simulink model "MPC_FOC"  (R2021a)
settings: Solver=VariableStepAuto  StartTime=0.0  StopTime=2  RelTol=1e-3
undefined symbols (not defined in the file): C1, JL, JM, K1, sigbuilder_block
libraries: powerlib_extras x9, spsDCVoltageSourceLib x4, spsPermanentMagnetSynchronousMachineLib x4, spsUniversalBridgeLib x4, spspowerguiLib x4, simulink x3, spsVoltageMeasurementLib x3, pid_lib x1
(part 2 of 2)

== system MPC_FOC/FOC/SVPWM/XYZ Caculate ==
  Ualpha : Inport
  Ubeta : Inport  Port=2
  Ts : Inport  Port=3
  Udc : Inport  Port=4
  Add : Sum
  Add1 : Sum  Inputs=+-
  Gain : Gain  Gain=3/2
  Gain1 : Gain  Gain=sqrt(3)
  Gain2 : Gain  Gain=sqrt(3)/2
  Math Function : Math  Operator=reciprocal  SignedPower=on  SaturateOnIntegerOverflow=on
  Mux : Mux  Inputs=3
  Product{,1..3} (4 alike) : Product
  XYZ : Outport
  wires:
  Mux/1 -> XYZ/1
  Product2/1 -> Mux/2
  Add1/1 -> Product3/1
  Add/1 -> Product2/1
  Gain2/1 -> Add/1, Add1/1
  Gain/1 -> Add1/2, Add/2
  Product3/1 -> Mux/3
  Product/1 -> Product3/2, Product2/2, Product1/2
  Product1/1 -> Mux/1
  Gain1/1 -> Product1/1
  Math Function/1 -> Product/2
  Udc/1 -> Math Function/1
  Ts/1 -> Product/1
  Ubeta/1 -> Gain1/1, Gain2/1
  Ualpha/1 -> Gain/1

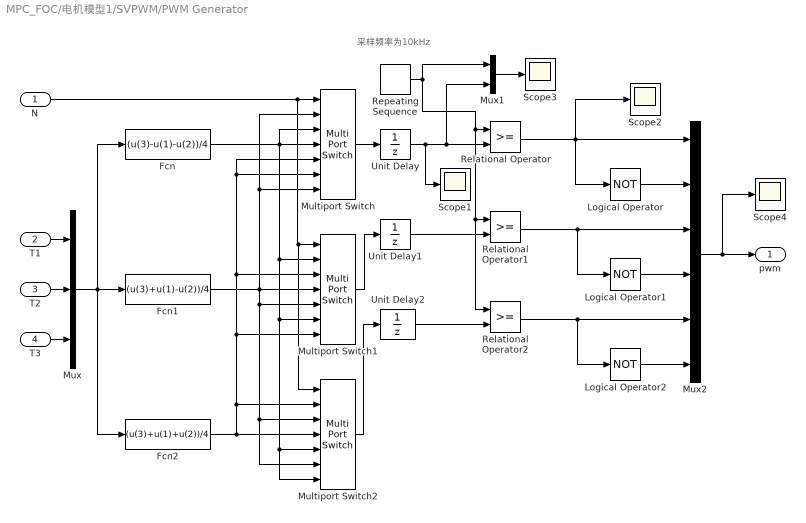
== system MPC_FOC/电机模型1/SVPWM/PWM Generator ==
  note: 采样频率为10kHz
  N : Inport
  T1 : Inport  Port=2
  T2 : Inport  Port=3
  T3 : Inport  Port=4
  Fcn : Fcn  Expr=(u(3)-u(1)-u(2))/4
  Fcn1 : Fcn  Expr=(u(3)+u(1)-u(2))/4
  Fcn2 : Fcn  Expr=(u(3)+u(1)+u(2))/4
  Logical Operator : Logic  Operator=NOT  AllPortsSameDT=off  OutDataTypeStr=boolean
  Logical Operator1 : Logic  Operator=NOT  AllPortsSameDT=off  OutDataTypeStr=boolean
  Logical Operator2 : Logic  Operator=NOT  AllPortsSameDT=off  OutDataTypeStr=boolean
  Multiport Switch : MultiPortSwitch  Inputs=6  DiagnosticForDefault=None
  Multiport Switch1 : MultiPortSwitch  Inputs=6  DiagnosticForDefault=None
  Multiport Switch2 : MultiPortSwitch  Inputs=6  DiagnosticForDefault=None
  Mux : Mux  Inputs=3
  Mux1 : Mux  Inputs=2
  Mux2 : Mux  Inputs=6
  Relational Operator : RelationalOperator  OutDataTypeStr=boolean  RndMeth=Nearest
  Relational Operator1 : RelationalOperator  OutDataTypeStr=boolean  RndMeth=Nearest
  Relational Operator2 : RelationalOperator  OutDataTypeStr=boolean  RndMeth=Nearest
  Repeating Sequence : simulink/Sources/Repeating Sequence  rep_seq_t=[0 0.00005 0.0001]  rep_seq_y=[0 0.00005 0]
  Scope{1..4} (4 alike) : Scope
  Unit Delay : UnitDelay  SampleTime=0.0001  HasFrameUpgradeWarning=on
  Unit Delay1 : UnitDelay  SampleTime=0.0001  HasFrameUpgradeWarning=on
  Unit Delay2 : UnitDelay  SampleTime=0.0001  HasFrameUpgradeWarning=on
  pwm : Outport
  wires:
  T2/1 -> Mux/2
  T1/1 -> Mux/1
  T3/1 -> Mux/3
  Mux/1 -> Fcn/1, Fcn1/1, Fcn2/1
  N/1 -> Multiport Switch2/1, Multiport Switch1/1, Multiport Switch/1
  Fcn/1 -> Multiport Switch2/7, Multiport Switch2/5, Multiport Switch1/6, Multiport Switch1/2, Multiport Switch/4, Multiport Switch/3
  Fcn1/1 -> Multiport Switch/7, Multiport Switch/2, Multiport Switch2/6, Multiport Switch2/3, Multiport Switch1/5, Multiport Switch1/4
  Fcn2/1 -> Multiport Switch2/4, Multiport Switch2/2, Multiport Switch1/7, Multiport Switch1/3, Multiport Switch/6, Multiport Switch/5
  Repeating Sequence/1 -> Mux1/1, Relational Operator2/1, Relational Operator1/1, Relational Operator/1
  Relational Operator/1 -> Scope2/1, Logical Operator/1, Mux2/1
  Relational Operator1/1 -> Logical Operator1/1, Mux2/3
  Relational Operator2/1 -> Logical Operator2/1, Mux2/5
  Logical Operator/1 -> Mux2/2
  Logical Operator1/1 -> Mux2/4
  Logical Operator2/1 -> Mux2/6
  Mux2/1 -> Scope4/1, pwm/1
  Multiport Switch1/1 -> Unit Delay1/1
  Multiport Switch2/1 -> Unit Delay2/1
  Multiport Switch/1 -> Unit Delay/1
  Mux1/1 -> Scope3/1
  Unit Delay/1 -> Mux1/2, Relational Operator/2, Scope1/1
  Unit Delay1/1 -> Relational Operator1/2
  Unit Delay2/1 -> Relational Operator2/2

== system MPC_FOC/电机模型1/SVPWM/Sector Caculate ==
  Ualpha : Inport
  "Ubeta " : Inport  Port=2
  Add : Sum  Inputs=+++
  Add1 : Sum  Inputs=+-
  Add2 : Sum  Inputs=--
  Constant : Constant
  Constant1 : Constant  Value=0
  Constant2 : Constant  Value=3/4
  Gain : Gain  Gain=4
  Gain1 : Gain  Gain=2
  Gain2 : Gain  Gain=0.5
  Product : Product
  Sqrt : Sqrt  SaturateOnIntegerOverflow=on
  Switch : Switch  Criteria=u2 > Threshold
  Switch1 : Switch  Criteria=u2 > Threshold
  Switch2 : Switch  Criteria=u2 > Threshold
  N : Outport
  wires:
  Ualpha/1 -> Product/1
  "Ubeta "/1 -> Switch/2, Gain2/1
  Add1/1 -> Switch1/2
  Add2/1 -> Switch2/2
  Constant/1 -> Switch/1, Switch1/1, Switch2/1
  Constant1/1 -> Switch2/3, Switch1/3, Switch/3
  Add/1 -> N/1
  Gain1/1 -> Add/2
  Gain/1 -> Add/3
  Switch2/1 -> Gain/1
  Switch1/1 -> Gain1/1
  Switch/1 -> Add/1
  Constant2/1 -> Sqrt/1
  Sqrt/1 -> Product/2
  Product/1 -> Add2/1, Add1/1
  Gain2/1 -> Add1/2, Add2/2

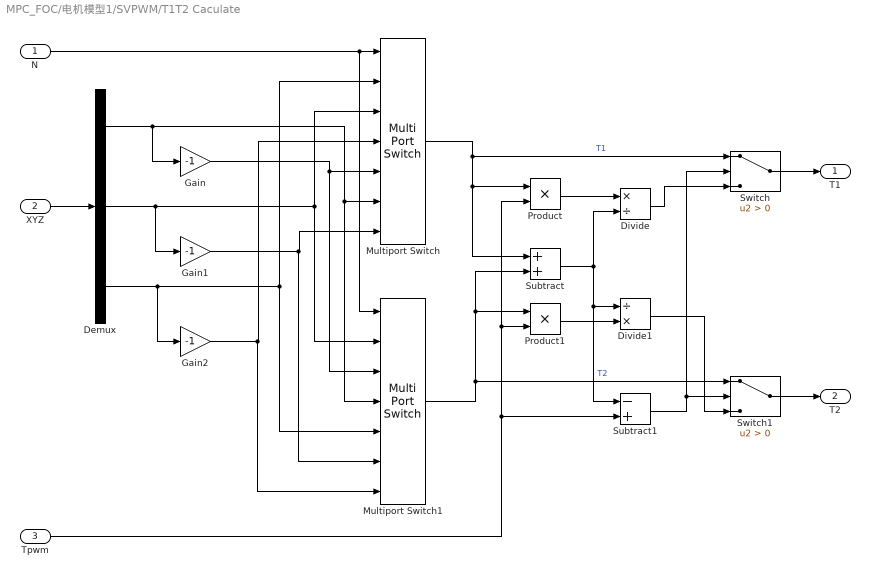
== system MPC_FOC/电机模型1/SVPWM/T1T2 Caculate ==
  N : Inport
  XYZ : Inport  Port=2
  Tpwm : Inport  Port=3
  Demux : Demux  Outputs=3
  Divide : Product  Inputs=*/
  Divide1 : Product  Inputs=/*
  Gain : Gain  Gain=-1
  Gain1 : Gain  Gain=-1
  Gain2 : Gain  Gain=-1
  Multiport Switch : MultiPortSwitch  Inputs=6  DiagnosticForDefault=None
  Multiport Switch1 : MultiPortSwitch  Inputs=6  DiagnosticForDefault=None
  Product : Product
  Product1 : Product
  Subtract : Sum
  Subtract1 : Sum  Inputs=-+
  Switch : Switch  Criteria=u2 > Threshold
  Switch1 : Switch  Criteria=u2 > Threshold
  "T1 " : Outport
  T2 : Outport  Port=2
  wires:
  N/1 -> Multiport Switch1/1, Multiport Switch/1
  Demux/1 -> Multiport Switch1/4, Multiport Switch/6, Gain/1
  Demux/2 -> Multiport Switch/3, Multiport Switch1/2, Gain1/1
  Demux/3 -> Gain2/1, Multiport Switch1/5, Multiport Switch/2
  Gain/1 -> Multiport Switch/5, Multiport Switch1/3
  Gain1/1 -> Multiport Switch1/6, Multiport Switch/7
  Gain2/1 -> Multiport Switch1/7, Multiport Switch/4
  XYZ/1 -> Demux/1
  Multiport Switch/1 -> Switch/1, Product/1, Subtract/1  "T1"
  Multiport Switch1/1 -> Subtract/2, Product1/1, Switch1/1  "T2"
  Tpwm/1 -> Subtract1/2, Product/2, Product1/2
  Divide/1 -> Switch/3
  Divide1/1 -> Switch1/3
  Subtract1/1 -> Switch1/2, Switch/2
  Switch1/1 -> T2/1
  Switch/1 -> "T1 "/1
  Product/1 -> Divide/1
  Subtract/1 -> Divide/2, Divide1/1, Subtract1/1
  Product1/1 -> Divide1/2

== system MPC_FOC/电机模型1/SVPWM/XYZ Caculate ==
  Ualpha : Inport
  Ubeta : Inport  Port=2
  Ts : Inport  Port=3
  Udc : Inport  Port=4
  Add : Sum
  Add1 : Sum  Inputs=+-
  Gain : Gain  Gain=3/2
  Gain1 : Gain  Gain=sqrt(3)
  Gain2 : Gain  Gain=sqrt(3)/2
  Math Function : Math  Operator=reciprocal  SignedPower=on  SaturateOnIntegerOverflow=on
  Mux : Mux  Inputs=3
  Product{,1..3} (4 alike) : Product
  XYZ : Outport
  wires:
  Ualpha/1 -> Gain/1
  Ubeta/1 -> Gain2/1, Gain1/1
  Ts/1 -> Product/1
  Udc/1 -> Math Function/1
  Math Function/1 -> Product/2
  Gain1/1 -> Product1/1
  Product1/1 -> Mux/1
  Product/1 -> Product1/2, Product2/2, Product3/2
  Product3/1 -> Mux/3
  Gain/1 -> Add/2, Add1/2
  Gain2/1 -> Add1/1, Add/1
  Add/1 -> Product2/1
  Add1/1 -> Product3/1
  Product2/1 -> Mux/2
  Mux/1 -> XYZ/1

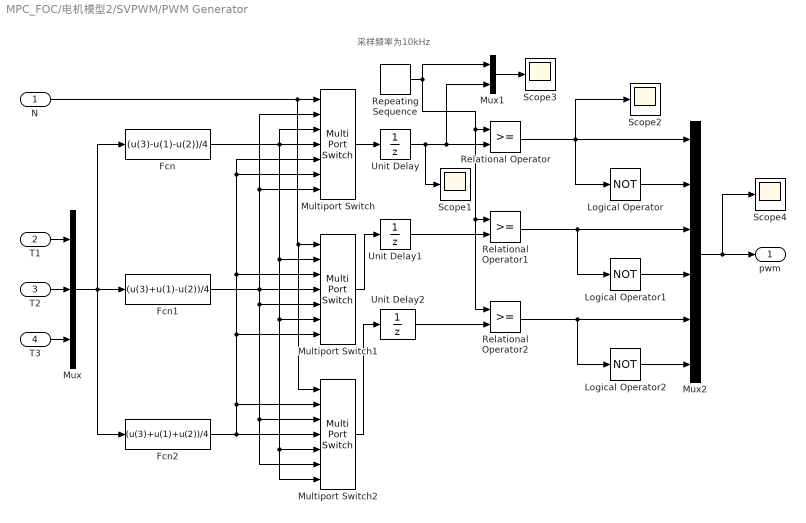
== system MPC_FOC/电机模型2/SVPWM/PWM Generator ==
  note: 采样频率为10kHz
  N : Inport
  T1 : Inport  Port=2
  T2 : Inport  Port=3
  T3 : Inport  Port=4
  Fcn : Fcn  Expr=(u(3)-u(1)-u(2))/4
  Fcn1 : Fcn  Expr=(u(3)+u(1)-u(2))/4
  Fcn2 : Fcn  Expr=(u(3)+u(1)+u(2))/4
  Logical Operator : Logic  Operator=NOT  AllPortsSameDT=off  OutDataTypeStr=boolean
  Logical Operator1 : Logic  Operator=NOT  AllPortsSameDT=off  OutDataTypeStr=boolean
  Logical Operator2 : Logic  Operator=NOT  AllPortsSameDT=off  OutDataTypeStr=boolean
  Multiport Switch : MultiPortSwitch  Inputs=6  DiagnosticForDefault=None
  Multiport Switch1 : MultiPortSwitch  Inputs=6  DiagnosticForDefault=None
  Multiport Switch2 : MultiPortSwitch  Inputs=6  DiagnosticForDefault=None
  Mux : Mux  Inputs=3
  Mux1 : Mux  Inputs=2
  Mux2 : Mux  Inputs=6
  Relational Operator : RelationalOperator  OutDataTypeStr=boolean  RndMeth=Nearest
  Relational Operator1 : RelationalOperator  OutDataTypeStr=boolean  RndMeth=Nearest
  Relational Operator2 : RelationalOperator  OutDataTypeStr=boolean  RndMeth=Nearest
  Repeating Sequence : simulink/Sources/Repeating Sequence  rep_seq_t=[0 0.00005 0.0001]  rep_seq_y=[0 0.00005 0]
  Scope{1..4} (4 alike) : Scope
  Unit Delay : UnitDelay  SampleTime=0.0001  HasFrameUpgradeWarning=on
  Unit Delay1 : UnitDelay  SampleTime=0.0001  HasFrameUpgradeWarning=on
  Unit Delay2 : UnitDelay  SampleTime=0.0001  HasFrameUpgradeWarning=on
  pwm : Outport
  wires:
  Unit Delay2/1 -> Relational Operator2/2
  Unit Delay1/1 -> Relational Operator1/2
  Unit Delay/1 -> Scope1/1, Relational Operator/2, Mux1/2
  Mux1/1 -> Scope3/1
  Multiport Switch/1 -> Unit Delay/1
  Multiport Switch2/1 -> Unit Delay2/1
  Multiport Switch1/1 -> Unit Delay1/1
  Mux2/1 -> pwm/1, Scope4/1
  Logical Operator2/1 -> Mux2/6
  Logical Operator1/1 -> Mux2/4
  Logical Operator/1 -> Mux2/2
  Relational Operator2/1 -> Mux2/5, Logical Operator2/1
  Relational Operator1/1 -> Mux2/3, Logical Operator1/1
  Relational Operator/1 -> Mux2/1, Logical Operator/1, Scope2/1
  Repeating Sequence/1 -> Relational Operator/1, Relational Operator1/1, Relational Operator2/1, Mux1/1
  Fcn2/1 -> Multiport Switch/5, Multiport Switch/6, Multiport Switch1/3, Multiport Switch1/7, Multiport Switch2/2, Multiport Switch2/4
  Fcn1/1 -> Multiport Switch1/4, Multiport Switch1/5, Multiport Switch2/3, Multiport Switch2/6, Multiport Switch/2, Multiport Switch/7
  Fcn/1 -> Multiport Switch/3, Multiport Switch/4, Multiport Switch1/2, Multiport Switch1/6, Multiport Switch2/5, Multiport Switch2/7
  N/1 -> Multiport Switch/1, Multiport Switch1/1, Multiport Switch2/1
  Mux/1 -> Fcn2/1, Fcn1/1, Fcn/1
  T3/1 -> Mux/3
  T1/1 -> Mux/1
  T2/1 -> Mux/2

== system MPC_FOC/电机模型2/SVPWM/Sector Caculate ==
  Ualpha : Inport
  "Ubeta " : Inport  Port=2
  Add : Sum  Inputs=+++
  Add1 : Sum  Inputs=+-
  Add2 : Sum  Inputs=--
  Constant : Constant
  Constant1 : Constant  Value=0
  Constant2 : Constant  Value=3/4
  Gain : Gain  Gain=4
  Gain1 : Gain  Gain=2
  Gain2 : Gain  Gain=0.5
  Product : Product
  Sqrt : Sqrt  SaturateOnIntegerOverflow=on
  Switch : Switch  Criteria=u2 > Threshold
  Switch1 : Switch  Criteria=u2 > Threshold
  Switch2 : Switch  Criteria=u2 > Threshold
  N : Outport
  wires:
  Gain2/1 -> Add2/2, Add1/2
  Product/1 -> Add1/1, Add2/1
  Sqrt/1 -> Product/2
  Constant2/1 -> Sqrt/1
  Switch/1 -> Add/1
  Switch1/1 -> Gain1/1
  Switch2/1 -> Gain/1
  Gain/1 -> Add/3
  Gain1/1 -> Add/2
  Add/1 -> N/1
  Constant1/1 -> Switch/3, Switch1/3, Switch2/3
  Constant/1 -> Switch2/1, Switch1/1, Switch/1
  Add2/1 -> Switch2/2
  Add1/1 -> Switch1/2
  "Ubeta "/1 -> Gain2/1, Switch/2
  Ualpha/1 -> Product/1

== system MPC_FOC/电机模型2/SVPWM/T1T2 Caculate ==
  N : Inport
  XYZ : Inport  Port=2
  Tpwm : Inport  Port=3
  Demux : Demux  Outputs=3
  Divide : Product  Inputs=*/
  Divide1 : Product  Inputs=/*
  Gain : Gain  Gain=-1
  Gain1 : Gain  Gain=-1
  Gain2 : Gain  Gain=-1
  Multiport Switch : MultiPortSwitch  Inputs=6  DiagnosticForDefault=None
  Multiport Switch1 : MultiPortSwitch  Inputs=6  DiagnosticForDefault=None
  Product : Product
  Product1 : Product
  Subtract : Sum
  Subtract1 : Sum  Inputs=-+
  Switch : Switch  Criteria=u2 > Threshold
  Switch1 : Switch  Criteria=u2 > Threshold
  "T1 " : Outport
  T2 : Outport  Port=2
  wires:
  Product1/1 -> Divide1/2
  Subtract/1 -> Subtract1/1, Divide1/1, Divide/2
  Product/1 -> Divide/1
  Switch/1 -> "T1 "/1
  Switch1/1 -> T2/1
  Subtract1/1 -> Switch/2, Switch1/2
  Divide1/1 -> Switch1/3
  Divide/1 -> Switch/3
  Tpwm/1 -> Product1/2, Product/2, Subtract1/2
  Multiport Switch1/1 -> Switch1/1, Product1/1, Subtract/2  "T2"
  Multiport Switch/1 -> Subtract/1, Product/1, Switch/1  "T1"
  XYZ/1 -> Demux/1
  Gain2/1 -> Multiport Switch/4, Multiport Switch1/7
  Gain1/1 -> Multiport Switch/7, Multiport Switch1/6
  Gain/1 -> Multiport Switch1/3, Multiport Switch/5
  Demux/3 -> Multiport Switch/2, Multiport Switch1/5, Gain2/1
  Demux/2 -> Gain1/1, Multiport Switch1/2, Multiport Switch/3
  Demux/1 -> Gain/1, Multiport Switch/6, Multiport Switch1/4
  N/1 -> Multiport Switch/1, Multiport Switch1/1

== system MPC_FOC/电机模型2/SVPWM/XYZ Caculate ==
  Ualpha : Inport
  Ubeta : Inport  Port=2
  Ts : Inport  Port=3
  Udc : Inport  Port=4
  Add : Sum
  Add1 : Sum  Inputs=+-
  Gain : Gain  Gain=3/2
  Gain1 : Gain  Gain=sqrt(3)
  Gain2 : Gain  Gain=sqrt(3)/2
  Math Function : Math  Operator=reciprocal  SignedPower=on  SaturateOnIntegerOverflow=on
  Mux : Mux  Inputs=3
  Product{,1..3} (4 alike) : Product
  XYZ : Outport
  wires:
  Mux/1 -> XYZ/1
  Product2/1 -> Mux/2
  Add1/1 -> Product3/1
  Add/1 -> Product2/1
  Gain2/1 -> Add/1, Add1/1
  Gain/1 -> Add1/2, Add/2
  Product3/1 -> Mux/3
  Product/1 -> Product3/2, Product2/2, Product1/2
  Product1/1 -> Mux/1
  Gain1/1 -> Product1/1
  Math Function/1 -> Product/2
  Udc/1 -> Math Function/1
  Ts/1 -> Product/1
  Ubeta/1 -> Gain1/1, Gain2/1
  Ualpha/1 -> Gain/1

== matlab function MPC_FOC/DVVMPC/2_vector_MPC_control1 ==
  settings: updateMethod=DISCRETE
  data: clock input; i_q_k input; i_d_k input; theta_e_r input; sa output; sb output; sc output; flux input; Ld input; Lq input; dtheta_e input; Te_k input; Te_ref input; phi_s_ref input
function [sa, sb, sc ] = fcn(clock, i_q_k, i_d_k, theta_e_r, flux, Ld, Lq, dtheta_e, Te_k, Te_ref, phi_s_ref)
%% 参数初始化
Ts = 0.0001;
cost = inf;
vdc = 400; % 定子电压
Rs = 0.11; % 电阻
pn = 4;
%% 获取控制周期内的相对时间
persistent time_start;
if isempty(time_start)
    time_start = clock;
end
time_relative = clock-time_start;
if time_relative >= Ts-1e-12
    time_start = clock;
    time_relative = 0;
end

%% 计算参考电压矢量
% % 无差拍控制下的phi_alpha\phi_beta
% ud_k = 0;
% ud_k = 0;
% i_d_k1 = (1-Rs*Ts/Ld)*i_d_k+Ts/Ld*(ud_k+dtheta_e*Lq*i_q_k);
% i_q_k1 = (1-Rs*Ts/Ld)*i_q_k+Ts/Ld*(uq_k-dtheta_e*Ld*i_d_k + dtheta_e*flux)

phi_dk = Ld*i_d_k +flux;
phi_qk = Lq*i_q_k;
X1 = phi_dk+dtheta_e*phi_qk*Ts;
B = ((2*Lq)/(3*pn*flux))*(Te_ref-Te_k) + (Rs*Ts*phi_qk)/Lq + dtheta_e*Ts*phi_dk;
X2 = B^2 + 2*B*(phi_qk-dtheta_e*phi_dk*Ts)+(1+dtheta_e^2*Ts^2)*(phi_dk^2+phi_qk^2) - phi_s_ref^2;
radicand = X1^2 - X2;
radicand = max(radicand, 1e-9);  % 限制最小值为1e-9，避免sqrt报错

ud_ref1 = (-X1 + sqrt(radicand)) / Ts;
ud_ref2 = (-X1 - sqrt(radicand)) / Ts;
% 选择幅值较小的解
if abs(ud_ref1) <= abs(ud_ref2)
    ud_ref = ud_ref1;
else
    ud_ref = ud_ref2;
end


uq_ref = B/Ts;
u_alpha_ref = cos(theta_e_r)*ud_ref - sin(theta_e_r)*uq_ref;
u_beta_ref = sin(theta_e_r)*ud_ref + cos(theta_e_r)*uq_ref;
theta_u_ref = atan2(u_beta_ref, u_alpha_ref);
if theta_u_ref<0
    theta_u_ref=theta_u_ref+2*pi;
end
%% 计算选择矢量
% 选择第一电压矢量
theta_norm_rel = theta_u_ref + pi/6;
if theta_norm_rel>2*pi
    theta_norm_rel=theta_norm_rel-2*pi;
end

sector = floor(theta_norm_rel / (pi/3)) + 1;
% 处理边界情况（刚好在扇区边界时归为当前扇区）
if sector == 7
    sector = 1;
end
voltage_vectors = [
    0 0 0;  % 0矢量V0
    1 0 0;  % 扇区1第一矢量V1
    1 1 0;  % 扇区2第一矢量V2
    0 1 0;  % 扇区3第一矢量V3
    0 1 1;  % 扇区4第一矢量V4
    0 0 1;  % 扇区5第一矢量V5
    1 0 1;  % 扇区6第一矢量V6
    1 1 1]; % 0矢量V7
% 选择当前扇区的第一电压矢量
first_vector = voltage_vectors(sector+1, :);
ua1 = first_vector(1)*vdc;
ub1 = first_vector(2)*vdc;
uc1 = first_vector(3)*vdc;
un1 = (ua1+ub1+uc1)/3;
u_an1 = ua1 - un1;
u_bn1 = ub1 - un1;
u_cn1 = uc1 - un1;
u_alpha_first = 2/3*(u_an1 - 1/2*u_bn1 - 1/2*u_cn1);
u_beta_first = 2/3*(sqrt(3)/2*u_bn1 - sqrt(3)/2*u_cn1);
% 选择第二电压矢量
% 开关次数约束
adjacent_sectors = {
    [7, 3, 1];  % 扇区1（V1）的相邻矢量：扇区2（V2）、扇区6（V6）
    [2, 4, 8];  % 扇区2（V2）的相邻矢量：扇区1（V1）、扇区3（V3）
    [3, 5, 1];  % 扇区3（V3）的相邻矢量：扇区2（V2）、扇区4（V4）
    [4, 6, 8];  % 扇区4（V4）的相邻矢量：扇区3（V3）、扇区5（V5）
    [5, 7, 1];  % 扇区5（V5）的相邻矢量：扇区4（V4）、扇区6（V6）
    [6, 2, 8]   % 扇区6（V6）的相邻矢量：扇区5（V5）、扇区1（V1）
    };
allowed_second_sectors = adjacent_sectors{sector};  % 允许的第二矢量sector

second_state = allowed_second_sectors(1);
for i = allowed_second_sectors
    second_vector = voltage_vectors(i,:);
    ua2 = second_vector(1)*vdc;
    ub2 = second_vector(2)*vdc;
    uc2 = second_vector(3)*vdc;
    un2 = (ua2+ub2+uc2)/3;
    u_an2 = ua2 - un2;
    u_bn2 = ub2 - un2;
    u_cn2 = uc2 - un2;
    u_alpha_second = 2/3*(u_an2 - 1/2*u_bn2 - 1/2*u_cn2);
    u_beta_second = 2/3*(sqrt(3)/2*u_bn2 - sqrt(3)/2*u_cn2);
    J = sqrt((u_alpha_ref-u_alpha_second)^2 + (u_beta_ref-u_beta_second)^2);
    if J<cost
        cost = J;
        second_state = i;
    end
    
end

second_vector = voltage_vectors(second_state, :);



%% 计算矢量作用时间
% αβ坐标系下参考电压矢量
% u_alpha_ref = Rs * i_alpha_k + (phi_alpha_k1 - phi_alpha_k)/Ts;
% u_beta_ref = Rs * i_beta_k + (phi_beta_k1 - phi_beta_k)/Ts;

% αβ坐标系下第一电压矢量
% u_alpha_first = 2/3*(u_an1 - 1/2*u_bn1 - 1/2*u_cn1);
% u_beta_first = 2/3*(sqrt(3)/2*u_bn1 - sqrt(3)/2*u_cn1);

% αβ坐标系下第二电压矢量
% u_alpha_second = 2/3*(u_an - 1/2*u_bn - 1/2*u_cn);
% u_beta_second = 2/3*(sqrt(3)/2*u_bn - sqrt(3)/2*u_cn);
num1 = (u_alpha_ref-u_alpha_second)*(u_alpha_first-u_alpha_second)+(u_beta_ref-u_beta_second)*(u_beta_first-u_beta_second);
num2 = (u_alpha_second-u_alpha_first)^2+(u_beta_second-u_beta_first)^2;
% num1 = u_alpha_ref*u_alpha_first + u_beta_ref*u_beta_first;
% num2 = u_alpha_ref^2+u_beta_ref^2;

t_1opt = num1/num2;

if t_1opt>1 
    t_1opt = 1;
end
if t_1opt<0
    t_1opt = 0;
end
% t_2opt = Ts - t_1opt;



%% 输出矢量
if time_relative < t_1opt*Ts-1e-12
%if time_relative < 2*Ts-1e-12
    sa = first_vector(1);
    sb = first_vector(2);
    sc = first_vector(3);

else
    sa = second_vector(1);
    sb = second_vector(2);
    sc = second_vector(3);    

end

== matlab function MPC_FOC/MPC_controller ==
  data: u output; thetaM_thetaL input; dthetaM_dthetaLL input; TM input; TL input; ref input
function u = mpc_controller3(thetaM_thetaL, dthetaM_dthetaLL, TM, TL, ref)
    % MPC控制器实现
    % 输入:
    %   y      - 当前系统输出
    %   r      - 参考输入(设定值)
    %   x  - 系统状态值 [dtheta1; dtheta3; dtheta2; theta1-theta2; thta1/i-theta3; TL; TM]
    %   Ts     - 采样时间
    % 输出:
    %   u      - 控制输出
    % --------------------------
    % 1. MPC参数设置
    % --------------------------
    x_hat = [thetaM_thetaL; dthetaM_dthetaLL; TM; TL];
    Np = 10;          % 预测时域
    Nc = 1;           % 控制时域
    u_min=0;
    u_max=20;
    % 设计权重矩阵
    Q = 102*eye(Np,Np);  % 状态权重矩阵
    R = 0.01;          % 控制输入权重
    Ts = 1e-5;
    %u_min = ;       % 控制输入下限
    %u_max = ;       % 控制输入上限
    %模型参数
    K1=10000;
    C1=2;
    JM=0.04;
    JL=0.1;
    i= 1;

    
    % --------------------------
    % 2. 系统模型离散化 (二阶系统)
    %    状态方程: dx/dt = Ax + Bu, y = Cx
    %    若Ts=1,离散状态方程：x(k+1)=Ts*(A+I)x(k) + Ts*Bu(k)
    % --------------------------
    A_cont = [
    0   1   0   0;                                             % 第1行
    -K1/JM-K1/JL   -C1/JM-C1/JL   1/JM  1/JL;                          % 第2行
    0  0  0  0;                                                  % 第3行
    0  0  0  0;                                                  % 第4行
    ]; % 连续时间状态矩阵
    B_cont = [0; 1/JM; 0; 0];          % 连续时间输入矩阵
    C_cont = [0 1 0 0];                % 输出矩阵
    I = eye(4,4);
    % 利用零阶保持器进行离散化
    %[A, B, C, ~] = c2d(A_cont, B_cont, C, 0, Ts);
    
    %前向欧拉法离散化
    A = Ts*A_cont+I;
    B = Ts*B_cont;
    C = C_cont;
    
    
    % --------------------------
    % 3. 构建预测模型 (状态空间形式)
    % --------------------------
    % 初始化预测矩阵
    Phi = zeros(Np*size(C,1), size(A,1));
    Gamma = zeros(Np*size(C,1), Nc);
    
    % 填充预测矩阵
    for m = 1:Np
        row_idx = (m-1)*size(C,1) + 1 : m*size(C,1);
        Phi(row_idx, :) = C*A^m;
        
        for n = 1:min(m, Nc)
            Gamma(row_idx, n) = C*A^(m-n)*B;
        end
    end
    
    % --------------------------
    % 4. 生成参考轨迹
    % --------------------------
    % 假设参考轨迹在预测时域内保持恒定
    
    
    % --------------------------
    % 5. 构建优化问题
    %    目标: min J = (Y - Y_ref)'Q_total(Y - Y_ref) + U'R_totalU
    % --------------------------
    % 构建权重矩阵
    
    
    
    
    
    % 计算跟踪误差：预测输出Y = Phi*x_hat + Gamma*U，误差 = Y - Y_ref
    Y_ref = repmat(ref, Np, 1);  % 扩展为Np×1向量（2×1）
    Y_pred = Phi * x_hat;
    
    tracking_error = Y_pred - Y_ref;  % 2x1误差向量（Np=2，n_y=1）
    
    % 修正线性项f（需转置为列向量，匹配quadprog要求）
    f = tracking_error' * Q * Gamma;  % 1xNc（Nc=1，故1x1）
    f = f';  % 转置为Nc×1列向量（1x1）
    
    % 修正二次项H（确保为Nc×Nc矩阵，R需扩展为对角矩阵）
    H = Gamma' * Q * Gamma + R * eye(Nc);  % 1x1矩阵（Nc=1）
    
    % 设置约束
    lb = repmat(u_min, Nc, 1);  % 控制输入下限
    %ub = repmat(u_max, Nc, 1);  % 控制输入上限
    
    % --------------------------
    % 6. 求解二次规划问题
    % --------------------------
    % 设置quadprog选项（指定算法为active-set）
    options = optimoptions('quadprog', ...
        'Display', 'off', ...
        'Algorithm', 'active-set', ...  % 必须指定，解决报错
        'MaxIterations', 1e3);
    % 求解优化问题
    %J_min = 0.5*U'*H*U+x_hat'*E*U;
    x0 = zeros(Nc, 1);  % Nc是控制时域，如Nc=1时x0=[0]，Nc=2时x0=[0;0]
    U = quadprog(H, f, [], [], [], [], [], [], x0, options);
    
    % --------------------------
    % 7. 应用第一个控制量 (滚动优化)
    % --------------------------
    u = U(1);
    % 防止控制量超出范围 (二次规划求解可能因数值问题略微超出)
    %u = max(min(u, u_max), u_min);
end

== matlab function MPC_FOC/DVVMPC/MTPA ==
  data: Te input; phi_s_ref output; Pn input; flux input; Ld input; Lq input; ita_ref output
function [phi_s_ref, ita_ref] = fcn(Te, Pn, flux, Ld, Lq)
%% MPTA原则计算phi_s_ref和ita_ref
% 对于表贴式PMSM (Ld = Lq)，MPTA条件就是id=0控制

% 计算q轴电流参考（id_ref = 0）
iq_ref = Te / (1.5 * Pn * flux);

% 计算定子磁链参考值
% phi_d = flux + Ld * id_ref = flux
% phi_q = Lq * iq_ref
phi_d_ref = flux;      % id=0
phi_q_ref = Lq * iq_ref;

phi_s_ref = sqrt(phi_d_ref^2 + phi_q_ref^2);

% 计算定子磁链参考角度
if abs(Te) < 1e-6
    ita_ref = 0;  % 零转矩时角度为0
else
    ita_ref = atan2(phi_q_ref, phi_d_ref);
end

% 确保角度在合理范围内
ita_ref = real(ita_ref);  % 避免复数
end

== matlab function MPC_FOC/DVVMPC/phi_s_k ==
  data: id_k input; phi_s_k output; iq_k input; flux input; Ld input; Lq input; ita_k output
function [phi_s_k,ita_k]  = fcn(id_k,iq_k,flux,Ld,Lq)
phi_q_k = Lq*iq_k;
phi_d_k = Ld*id_k + flux;
phi_s_k = sqrt(phi_q_k^2+phi_d_k^2);
ita_k = atan2(phi_q_k, phi_d_k);

end
